simulink library "HS_lib"  (R2024a)
settings: Solver=VariableStepAuto  StartTime=0.0  StopTime=10.0  RelTol=1e-3
settings Model: Creator=Anna  LastModifiedBy=Anna

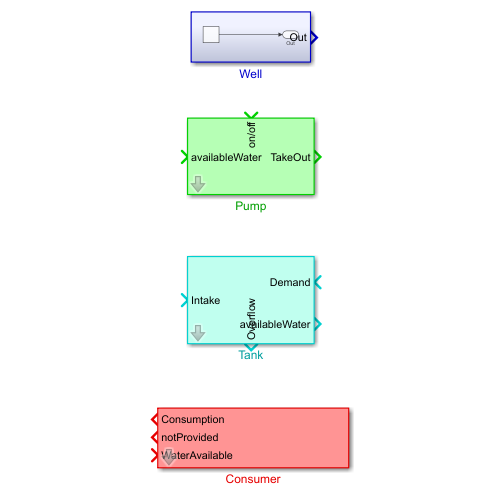
[thumbnail: Simulink's stored preview of the top-level diagram]
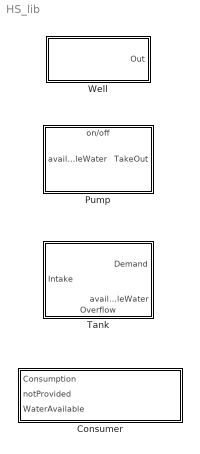
== system HS_lib ==
  Consumer : Subsystem  mask{d=0, a=0, f=0}
      mask prompts: d "Delay"; a "Amplitude"; f "Frequency"
      settings: PortSchema="{\"entries\":[{\"content\":{\"sides\":[{\"content\":{\"connectorIds\":[\"Out1\",\"Out2\",\"In1\"]},\"type\":\"ConnectorPlacement.EquallySpacedRectSide\",\"uuid\":\"64b5a97a-4244-4f26-899d-15714f2aa8f6\"},{\"content\":{\"side\":\"RIGHT\"},\"type\":\"ConnectorPlacement.EquallySpacedRectSide\",\"uuid\":\"d3b45f67-9c9d-4eef-86a5-95557b8542c4\"},{\"content\":{\"side\":\"TOP\"},\"type\":\"ConnectorPlacement.EquallySpacedRectSide\",\"uuid\":\"2b7281c0-f61f-45e3-808b-a4fd1d62cbbb\"}]},\"type\":\"ConnectorPlacement.EquallySpacedConnector\",\"uuid\":\"1937d4df-e955-4a14-a18e-eb0cc3956b4d\"}],\"packageUris\":[\"http://schema.mathworks.com/mf0/Connector/R2020b\"],\"version\":\"1.0\"}"
  Pump : Subsystem  mask{p=0}
      mask prompts: p "Power"
      settings: PortSchema="{\"entries\":[{\"content\":{\"sides\":[{\"content\":{\"connectorIds\":[\"In1\"]},\"type\":\"ConnectorPlacement.EquallySpacedRectSide\",\"uuid\":\"19044534-5fed-425e-9b28-cfa8ce8c2d07\"},{\"content\":{\"connectorIds\":[\"Out1\"],\"side\":\"RIGHT\"},\"type\":\"ConnectorPlacement.EquallySpacedRectSide\",\"uuid\":\"25083535-857b-4aa6-b643-c29d52fd8b89\"},{\"content\":{\"connectorIds\":[\"In2\"],\"side\":\"TOP\"},\"type\":\"ConnectorPlacement.EquallySpacedRectSide\",\"uuid\":\"599575d0-15e5-44fc-9209-be917a93ad07\"}]},\"type\":\"ConnectorPlacement.EquallySpacedConnector\",\"uuid\":\"7a1b4f14-afb7-42e2-aa80-653c0fb5067f\"}],\"packageUris\":[\"http://schema.mathworks.com/mf0/Connector/R2020b\"],\"version\":\"1.0\"}"
  Tank : Subsystem  mask{c_init=0, c=100}
      mask prompts: c_init "initial Capacity"; c "Capacity"
      settings: PortSchema="{\"entries\":[{\"content\":{\"sides\":[{\"content\":{\"connectorIds\":[\"In1\"]},\"type\":\"ConnectorPlacement.EquallySpacedRectSide\",\"uuid\":\"19044534-5fed-425e-9b28-cfa8ce8c2d07\"},{\"content\":{\"connectorIds\":[\"In2\",\"Out1\"],\"side\":\"RIGHT\"},\"type\":\"ConnectorPlacement.EquallySpacedRectSide\",\"uuid\":\"25083535-857b-4aa6-b643-c29d52fd8b89\"},{\"content\":{\"side\":\"TOP\"},\"type\":\"ConnectorPlacement.EquallySpacedRectSide\",\"uuid\":\"599575d0-15e5-44fc-9209-be917a93ad07\"},{\"content\":{\"connectorIds\":[\"Out2\"],\"side\":\"BOTTOM\"},\"type\":\"ConnectorPlacement.EquallySpacedRectSide\",\"uuid\":\"799f4d24-f4f0-4738-a8a2-f0c8281d36dc\"}]},\"type\":\"ConnectorPlacement.EquallySpacedConnector\",\"uuid\":\"7a1b4f14-afb7-42e2-aa80-653c0fb5067f\"}],\"packageUris\":[\"http://schema.mathworks.com/mf0/Connector/R2020b\"],\"version\":\"1.0\"}"
  Well : Subsystem

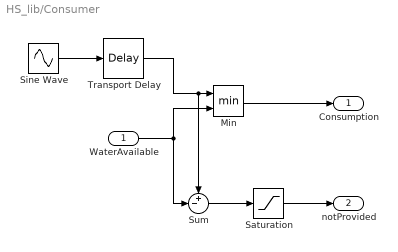
== system HS_lib/Consumer ==
  WaterAvailable : Inport
  Min : MinMax  Inputs=2
  Saturation : Saturate  UpperLimit=inf  LowerLimit=0
  Sine Wave : Sin  Amplitude=a  Bias=a  Frequency=f  SampleTime=0
  Sum : Sum  Inputs=+-|
  Transport Delay : TransportDelay  DelayTime=d  InitialOutput=a
  Consumption : Outport
  notProvided : Outport  Port=2
  wires:
  WaterAvailable/1 -> Sum/2, Min/2
  Min/1 -> Consumption/1
  Transport Delay/1 -> Sum/1, Min/1
  Sine Wave/1 -> Transport Delay/1
  Sum/1 -> Saturation/1
  Saturation/1 -> notProvided/1

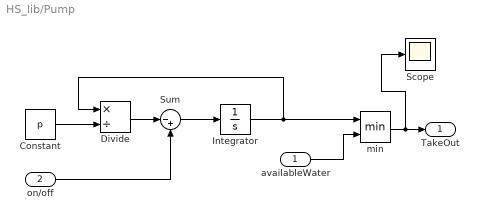
== system HS_lib/Pump ==
  availableWater : Inport
  on/off : Inport  Port=2  OutDataTypeStr=boolean
  Constant : Constant  Value=p
  Divide : Product  Inputs=*/
  Integrator : Integrator
  Scope : Scope
  Sum : Sum  Inputs=|-+
  min : MinMax  Inputs=2
  TakeOut : Outport
  wires:
  min/1 -> TakeOut/1, Scope/1
  availableWater/1 -> min/2
  Divide/1 -> Sum/1
  Constant/1 -> Divide/2
  Integrator/1 -> min/1, Divide/1
  Sum/1 -> Integrator/1
  on/off/1 -> Sum/2

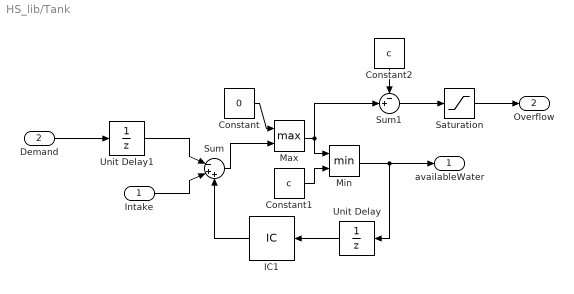
== system HS_lib/Tank ==
  Intake : Inport
  Demand : Inport  Port=2
  Constant : Constant  Value=0
  Constant1 : Constant  Value=c
  Constant2 : Constant  Value=c
  IC1 : InitialCondition  Value=c_init
  Max : MinMax  Function=max  Inputs=2
  Min : MinMax  Inputs=2
  Saturation : Saturate  UpperLimit=inf  LowerLimit=0
  Sum : Sum  Inputs=|-++
  Sum1 : Sum  Inputs=-+|
  Unit Delay : UnitDelay  SampleTime=-1  HasFrameUpgradeWarning=on
  Unit Delay1 : UnitDelay  SampleTime=-1  HasFrameUpgradeWarning=on
  availableWater : Outport
  Overflow : Outport  Port=2
  wires:
  Saturation/1 -> Overflow/1
  Constant2/1 -> Sum1/1
  Unit Delay1/1 -> Sum/1
  Unit Delay/1 -> IC1/1
  Sum1/1 -> Saturation/1
  Min/1 -> availableWater/1, Unit Delay/1
  Constant1/1 -> Min/2
  Max/1 -> Min/1, Sum1/2
  Constant/1 -> Max/1
  IC1/1 -> Sum/3
  Sum/1 -> Max/2
  Demand/1 -> Unit Delay1/1
  Intake/1 -> Sum/2

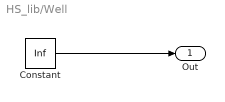
== system HS_lib/Well ==
  Constant : Constant  Value=Inf
  Out : Outport
  wires:
  Constant/1 -> Out/1
